simulink library "halout"  (R2021b)
settings: Solver=VariableStepAuto  StartTime=0.0  StopTime=10.0  RelTol=1e-3
undefined symbols (not defined in the file): C_TASK_5MS_S, FALSE, KHAL_CAN1FD1APS3E2E_flg, KHAL_CAN1FD1APS3TxReq_flg, KHAL_CAN1FD1VCU2E2E_flg, KHAL_CAN1FD1VCU2TxReq_flg, KHAL_CAN1FD1VCU3E2E_flg, KHAL_CAN1FD1VCU3TxReq_flg, KHAL_CAN1TxReq_flg, KHAL_CAN1VMCFCM1E2E_flg, KHAL_CAN1VMCFCM1TxReq_flg, KHAL_CAN2TxReq_flg, KHAL_CAN3FD3VCU1toNIDECTxReq_flg, KHAL_CAN3FD3VCU1TxReq_flg, KHAL_CAN3FD3VCU2E2E_flg, KHAL_CAN3FD3VCU2toNIDECE2E_flg, KHAL_CAN3FD3VCU2toNIDECTxReq_flg, KHAL_CAN3FD3VCU2TxReq_flg, KHAL_CAN3TxReq_flg, KHAL_CAN4FD4CE1000E2E_flg, KHAL_CAN4FD4CE1000TxReq_flg, KHAL_CAN4TxReq_flg, KHAL_CAN5TxReq_flg, KHAL_CAN6FD6APS3E2E_flg, KHAL_CAN6FD6APS3TxReq_flg, KHAL_CAN6FD6VCU2E2E_flg, KHAL_CAN6FD6VCU2TxReq_flg, KHAL_CAN6TxReq_flg, ONE_INT, TRUE, ZERO_INT
libraries: FVT_lib x500, simulink x235
(part 18 of 25)

== system halout/HAL_OUT/CAN2/FD2_CE200_1_0x435/LFWheelPress ==
  LFWheelPress : Inport
  Data Type Conversion : DataTypeConversion  OutDataTypeStr=uint8  RndMeth=Round
  CAN2_LFWheelPress : Outport
  wires:
  Data Type Conversion/1 -> CAN2_LFWheelPress/1
  LFWheelPress/1 -> Data Type Conversion/1

== system halout/HAL_OUT/CAN2/FD2_CE200_1_0x435/LFWheelShield ==
  LFWheelShield : Inport
  Data Type Conversion : DataTypeConversion  OutDataTypeStr=uint8  RndMeth=Round
  CAN2_LFWheelShield : Outport
  wires:
  Data Type Conversion/1 -> CAN2_LFWheelShield/1
  LFWheelShield/1 -> Data Type Conversion/1

== system halout/HAL_OUT/CAN2/FD2_CE200_1_0x435/LFWheelTemp ==
  LFWheelTemp : Inport
  Data Type Conversion : DataTypeConversion  OutDataTypeStr=uint8  RndMeth=Round
  convert_out : FVT_lib/hal/convert_out  gain=1  offset=-40
  CAN2_LFWheelTemp : Outport
  wires:
  Data Type Conversion/1 -> CAN2_LFWheelTemp/1
  convert_out/1 -> Data Type Conversion/1
  LFWheelTemp/1 -> convert_out/1

== system halout/HAL_OUT/CAN2/FD2_CE200_1_0x435/LFWheelTmpIndi ==
  LFWheelTmpIndi : Inport
  Data Type Conversion : DataTypeConversion  OutDataTypeStr=uint8  RndMeth=Round
  CAN2_LFWheelTmpIndi : Outport
  wires:
  Data Type Conversion/1 -> CAN2_LFWheelTmpIndi/1
  LFWheelTmpIndi/1 -> Data Type Conversion/1

== system halout/HAL_OUT/CAN2/FD2_CE200_1_0x435/LRBatWarn ==
  LRBatWarn : Inport
  Data Type Conversion : DataTypeConversion  OutDataTypeStr=uint8  RndMeth=Round
  CAN2_LRBatWarn : Outport
  wires:
  Data Type Conversion/1 -> CAN2_LRBatWarn/1
  LRBatWarn/1 -> Data Type Conversion/1

== system halout/HAL_OUT/CAN2/FD2_CE200_1_0x435/LRPressIndi ==
  LRPressIndi : Inport
  Data Type Conversion : DataTypeConversion  OutDataTypeStr=uint8  RndMeth=Round
  CAN2_LRPressIndi : Outport
  wires:
  Data Type Conversion/1 -> CAN2_LRPressIndi/1
  LRPressIndi/1 -> Data Type Conversion/1

== system halout/HAL_OUT/CAN2/FD2_CE200_1_0x435/LRSensorFail ==
  LRSensorFail : Inport
  Data Type Conversion : DataTypeConversion  OutDataTypeStr=uint8  RndMeth=Round
  CAN2_LRSensorFail : Outport
  wires:
  Data Type Conversion/1 -> CAN2_LRSensorFail/1
  LRSensorFail/1 -> Data Type Conversion/1

== system halout/HAL_OUT/CAN2/FD2_CE200_1_0x435/LRWheelDebug ==
  LRWheelDebug : Inport
  Data Type Conversion : DataTypeConversion  OutDataTypeStr=uint8  RndMeth=Round
  CAN2_LRWheelDebug : Outport
  wires:
  Data Type Conversion/1 -> CAN2_LRWheelDebug/1
  LRWheelDebug/1 -> Data Type Conversion/1

== system halout/HAL_OUT/CAN2/FD2_CE200_1_0x435/LRWheelPSW ==
  LRWheelPSW : Inport
  Data Type Conversion : DataTypeConversion  OutDataTypeStr=uint8  RndMeth=Round
  CAN2_LRWheelPSW : Outport
  wires:
  Data Type Conversion/1 -> CAN2_LRWheelPSW/1
  LRWheelPSW/1 -> Data Type Conversion/1

== system halout/HAL_OUT/CAN2/FD2_CE200_1_0x435/LRWheelPress ==
  LRWheelPress : Inport
  Data Type Conversion : DataTypeConversion  OutDataTypeStr=uint8  RndMeth=Round
  CAN2_LRWheelPress : Outport
  wires:
  Data Type Conversion/1 -> CAN2_LRWheelPress/1
  LRWheelPress/1 -> Data Type Conversion/1

== system halout/HAL_OUT/CAN2/FD2_CE200_1_0x435/LRWheelShield ==
  LRWheelShield : Inport
  Data Type Conversion : DataTypeConversion  OutDataTypeStr=uint8  RndMeth=Round
  CAN2_LRWheelShield : Outport
  wires:
  Data Type Conversion/1 -> CAN2_LRWheelShield/1
  LRWheelShield/1 -> Data Type Conversion/1

== system halout/HAL_OUT/CAN2/FD2_CE200_1_0x435/LRWheelTemp ==
  LRWheelTemp : Inport
  Data Type Conversion : DataTypeConversion  OutDataTypeStr=uint8  RndMeth=Round
  convert_out : FVT_lib/hal/convert_out  gain=1  offset=-40
  CAN2_LRWheelTemp : Outport
  wires:
  Data Type Conversion/1 -> CAN2_LRWheelTemp/1
  convert_out/1 -> Data Type Conversion/1
  LRWheelTemp/1 -> convert_out/1

== system halout/HAL_OUT/CAN2/FD2_CE200_1_0x435/LRWheelTmpIndi ==
  LRWheelTmpIndi : Inport
  Data Type Conversion : DataTypeConversion  OutDataTypeStr=uint8  RndMeth=Round
  CAN2_LRWheelTmpIndi : Outport
  wires:
  Data Type Conversion/1 -> CAN2_LRWheelTmpIndi/1
  LRWheelTmpIndi/1 -> Data Type Conversion/1

== system halout/HAL_OUT/CAN2/FD2_CE200_1_0x435/RFBatWarn ==
  RFBatWarn : Inport
  Data Type Conversion : DataTypeConversion  OutDataTypeStr=uint8  RndMeth=Round
  CAN2_RFBatWarn : Outport
  wires:
  Data Type Conversion/1 -> CAN2_RFBatWarn/1
  RFBatWarn/1 -> Data Type Conversion/1

== system halout/HAL_OUT/CAN2/FD2_CE200_1_0x435/RFPressIndi ==
  RFPressIndi : Inport
  Data Type Conversion : DataTypeConversion  OutDataTypeStr=uint8  RndMeth=Round
  CAN2_RFPressIndi : Outport
  wires:
  Data Type Conversion/1 -> CAN2_RFPressIndi/1
  RFPressIndi/1 -> Data Type Conversion/1

== system halout/HAL_OUT/CAN2/FD2_CE200_1_0x435/RFSensorFail ==
  RFSensorFail : Inport
  Data Type Conversion : DataTypeConversion  OutDataTypeStr=uint8  RndMeth=Round
  CAN2_RFSensorFail : Outport
  wires:
  Data Type Conversion/1 -> CAN2_RFSensorFail/1
  RFSensorFail/1 -> Data Type Conversion/1

== system halout/HAL_OUT/CAN2/FD2_CE200_1_0x435/RFWheelDebug ==
  RFWheelDebug : Inport
  Data Type Conversion : DataTypeConversion  OutDataTypeStr=uint8  RndMeth=Round
  CAN2_RFWheelDebug : Outport
  wires:
  Data Type Conversion/1 -> CAN2_RFWheelDebug/1
  RFWheelDebug/1 -> Data Type Conversion/1

== system halout/HAL_OUT/CAN2/FD2_CE200_1_0x435/RFWheelPSW ==
  RFWheelPSW : Inport
  Data Type Conversion : DataTypeConversion  OutDataTypeStr=uint8  RndMeth=Round
  CAN2_RFWheelPSW : Outport
  wires:
  Data Type Conversion/1 -> CAN2_RFWheelPSW/1
  RFWheelPSW/1 -> Data Type Conversion/1

== system halout/HAL_OUT/CAN2/FD2_CE200_1_0x435/RFWheelPress ==
  RFWheelPress : Inport
  Data Type Conversion : DataTypeConversion  OutDataTypeStr=uint8  RndMeth=Round
  CAN2_RFWheelPress : Outport
  wires:
  Data Type Conversion/1 -> CAN2_RFWheelPress/1
  RFWheelPress/1 -> Data Type Conversion/1

== system halout/HAL_OUT/CAN2/FD2_CE200_1_0x435/RFWheelShield ==
  RFWheelShield : Inport
  Data Type Conversion : DataTypeConversion  OutDataTypeStr=uint8  RndMeth=Round
  CAN2_RFWheelShield : Outport
  wires:
  Data Type Conversion/1 -> CAN2_RFWheelShield/1
  RFWheelShield/1 -> Data Type Conversion/1

== system halout/HAL_OUT/CAN2/FD2_CE200_1_0x435/RFWheelTemp ==
  RFWheelTemp : Inport
  Data Type Conversion : DataTypeConversion  OutDataTypeStr=uint8  RndMeth=Round
  convert_out : FVT_lib/hal/convert_out  gain=1  offset=-40
  CAN2_RFWheelTemp : Outport
  wires:
  Data Type Conversion/1 -> CAN2_RFWheelTemp/1
  convert_out/1 -> Data Type Conversion/1
  RFWheelTemp/1 -> convert_out/1

== system halout/HAL_OUT/CAN2/FD2_CE200_1_0x435/RFWheelTmpIndi ==
  RFWheelTmpIndi : Inport
  Data Type Conversion : DataTypeConversion  OutDataTypeStr=uint8  RndMeth=Round
  CAN2_RFWheelTmpIndi : Outport
  wires:
  Data Type Conversion/1 -> CAN2_RFWheelTmpIndi/1
  RFWheelTmpIndi/1 -> Data Type Conversion/1

== system halout/HAL_OUT/CAN2/FD2_CE200_1_0x435/RRBatWarn ==
  RRBatWarn : Inport
  Data Type Conversion : DataTypeConversion  OutDataTypeStr=uint8  RndMeth=Round
  CAN2_RRBatWarn : Outport
  wires:
  Data Type Conversion/1 -> CAN2_RRBatWarn/1
  RRBatWarn/1 -> Data Type Conversion/1

== system halout/HAL_OUT/CAN2/FD2_CE200_1_0x435/RRPressIndi ==
  RRPressIndi : Inport
  Data Type Conversion : DataTypeConversion  OutDataTypeStr=uint8  RndMeth=Round
  CAN2_RRPressIndi : Outport
  wires:
  Data Type Conversion/1 -> CAN2_RRPressIndi/1
  RRPressIndi/1 -> Data Type Conversion/1

== system halout/HAL_OUT/CAN2/FD2_CE200_1_0x435/RRSensorFail ==
  RRSensorFail : Inport
  Data Type Conversion : DataTypeConversion  OutDataTypeStr=uint8  RndMeth=Round
  CAN2_RRSensorFail : Outport
  wires:
  Data Type Conversion/1 -> CAN2_RRSensorFail/1
  RRSensorFail/1 -> Data Type Conversion/1

== system halout/HAL_OUT/CAN2/FD2_CE200_1_0x435/RRWheelDebug ==
  RRWheelDebug : Inport
  Data Type Conversion : DataTypeConversion  OutDataTypeStr=uint8  RndMeth=Round
  CAN2_RRWheelDebug : Outport
  wires:
  Data Type Conversion/1 -> CAN2_RRWheelDebug/1
  RRWheelDebug/1 -> Data Type Conversion/1

== system halout/HAL_OUT/CAN2/FD2_CE200_1_0x435/RRWheelPSW ==
  RRWheelPSW : Inport
  Data Type Conversion : DataTypeConversion  OutDataTypeStr=uint8  RndMeth=Round
  CAN2_RRWheelPSW : Outport
  wires:
  Data Type Conversion/1 -> CAN2_RRWheelPSW/1
  RRWheelPSW/1 -> Data Type Conversion/1

== system halout/HAL_OUT/CAN2/FD2_CE200_1_0x435/RRWheelPress ==
  RRWheelPress : Inport
  Data Type Conversion : DataTypeConversion  OutDataTypeStr=uint8  RndMeth=Round
  CAN2_RRWheelPress : Outport
  wires:
  Data Type Conversion/1 -> CAN2_RRWheelPress/1
  RRWheelPress/1 -> Data Type Conversion/1

== system halout/HAL_OUT/CAN2/FD2_CE200_1_0x435/RRWheelShield ==
  RRWheelShield : Inport
  Data Type Conversion : DataTypeConversion  OutDataTypeStr=uint8  RndMeth=Round
  CAN2_RRWheelShield : Outport
  wires:
  Data Type Conversion/1 -> CAN2_RRWheelShield/1
  RRWheelShield/1 -> Data Type Conversion/1

== system halout/HAL_OUT/CAN2/FD2_CE200_1_0x435/RRWheelTemp ==
  RRWheelTemp : Inport
  Data Type Conversion : DataTypeConversion  OutDataTypeStr=uint8  RndMeth=Round
  convert_out : FVT_lib/hal/convert_out  gain=1  offset=-40
  CAN2_RRWheelTemp : Outport
  wires:
  Data Type Conversion/1 -> CAN2_RRWheelTemp/1
  convert_out/1 -> Data Type Conversion/1
  RRWheelTemp/1 -> convert_out/1

== system halout/HAL_OUT/CAN2/FD2_CE200_1_0x435/RRWheelTmpIndi ==
  RRWheelTmpIndi : Inport
  Data Type Conversion : DataTypeConversion  OutDataTypeStr=uint8  RndMeth=Round
  CAN2_RRWheelTmpIndi : Outport
  wires:
  Data Type Conversion/1 -> CAN2_RRWheelTmpIndi/1
  RRWheelTmpIndi/1 -> Data Type Conversion/1

== system halout/HAL_OUT/CAN2/FD2_CE200_1_0x435/TPMSCaliButtAllow ==
  TPMSCaliButtAllow : Inport
  Data Type Conversion : DataTypeConversion  OutDataTypeStr=uint8  RndMeth=Round
  CAN2_TPMS_Cali_Butt_Allow : Outport
  wires:
  Data Type Conversion/1 -> CAN2_TPMS_Cali_Butt_Allow/1
  TPMSCaliButtAllow/1 -> Data Type Conversion/1

== system halout/HAL_OUT/CAN2/FD2_CE200_1_0x435/TPMSResButtAllow ==
  TPMSResButtAllow : Inport
  Data Type Conversion : DataTypeConversion  OutDataTypeStr=uint8  RndMeth=Round
  CAN2_TPMS_Res_Butt_Allow : Outport
  wires:
  Data Type Conversion/1 -> CAN2_TPMS_Res_Butt_Allow/1
  TPMSResButtAllow/1 -> Data Type Conversion/1

== system halout/HAL_OUT/CAN2/FD2_CE200_1_0x435/TPMSWarnIndi ==
  TPMSWarnIndi : Inport
  Data Type Conversion : DataTypeConversion  OutDataTypeStr=uint8  RndMeth=Round
  CAN2_TPMSWarnIndi : Outport
  wires:
  Data Type Conversion/1 -> CAN2_TPMSWarnIndi/1
  TPMSWarnIndi/1 -> Data Type Conversion/1

== system halout/HAL_OUT/CAN2/FD2_Version_0x3C3/FUSIONHWVer1 ==
  FUSIONHWVer1 : Inport
  Data Type Conversion : DataTypeConversion  OutDataTypeStr=uint8  RndMeth=Round
  CAN2_FUSION_HW_Ver1 : Outport
  wires:
  Data Type Conversion/1 -> CAN2_FUSION_HW_Ver1/1
  FUSIONHWVer1/1 -> Data Type Conversion/1

== system halout/HAL_OUT/CAN2/FD2_Version_0x3C3/FUSIONHWVer2 ==
  FUSIONHWVer2 : Inport
  Data Type Conversion : DataTypeConversion  OutDataTypeStr=uint8  RndMeth=Round
  CAN2_FUSION_HW_Ver2 : Outport
  wires:
  Data Type Conversion/1 -> CAN2_FUSION_HW_Ver2/1
  FUSIONHWVer2/1 -> Data Type Conversion/1

== system halout/HAL_OUT/CAN2/FD2_Version_0x3C3/FUSIONHWVer3 ==
  FUSIONHWVer3 : Inport
  Data Type Conversion : DataTypeConversion  OutDataTypeStr=uint8  RndMeth=Round
  CAN2_FUSION_HW_Ver3 : Outport
  wires:
  Data Type Conversion/1 -> CAN2_FUSION_HW_Ver3/1
  FUSIONHWVer3/1 -> Data Type Conversion/1

== system halout/HAL_OUT/CAN2/FD2_Version_0x3C3/FUSIONSWCarModel1 ==
  FUSIONSWCarModel1 : Inport
  Data Type Conversion : DataTypeConversion  OutDataTypeStr=uint8  RndMeth=Round
  CAN2_FUSION_SW_CarModel1 : Outport
  wires:
  Data Type Conversion/1 -> CAN2_FUSION_SW_CarModel1/1
  FUSIONSWCarModel1/1 -> Data Type Conversion/1

== system halout/HAL_OUT/CAN2/FD2_Version_0x3C3/FUSIONSWCarModel2 ==
  FUSIONSWCarModel2 : Inport
  Data Type Conversion : DataTypeConversion  OutDataTypeStr=uint8  RndMeth=Round
  CAN2_FUSION_SW_CarModel2 : Outport
  wires:
  Data Type Conversion/1 -> CAN2_FUSION_SW_CarModel2/1
  FUSIONSWCarModel2/1 -> Data Type Conversion/1

== system halout/HAL_OUT/CAN2/FD2_Version_0x3C3/FUSIONSWCarModel3 ==
  FUSIONSWCarModel3 : Inport
  Data Type Conversion : DataTypeConversion  OutDataTypeStr=uint8  RndMeth=Round
  CAN2_FUSION_SW_CarModel3 : Outport
  wires:
  Data Type Conversion/1 -> CAN2_FUSION_SW_CarModel3/1
  FUSIONSWCarModel3/1 -> Data Type Conversion/1

== system halout/HAL_OUT/CAN2/FD2_Version_0x3C3/FUSIONSWController1 ==
  FUSIONSWController1 : Inport
  Data Type Conversion : DataTypeConversion  OutDataTypeStr=uint8  RndMeth=Round
  CAN2_FUSION_SW_Controller1 : Outport
  wires:
  Data Type Conversion/1 -> CAN2_FUSION_SW_Controller1/1
  FUSIONSWController1/1 -> Data Type Conversion/1

== system halout/HAL_OUT/CAN2/FD2_Version_0x3C3/FUSIONSWController2 ==
  FUSIONSWController2 : Inport
  Data Type Conversion : DataTypeConversion  OutDataTypeStr=uint8  RndMeth=Round
  CAN2_FUSION_SW_Controller2 : Outport
  wires:
  Data Type Conversion/1 -> CAN2_FUSION_SW_Controller2/1
  FUSIONSWController2/1 -> Data Type Conversion/1

== system halout/HAL_OUT/CAN2/FD2_Version_0x3C3/FUSIONSWCountry1 ==
  FUSIONSWCountry1 : Inport
  Data Type Conversion : DataTypeConversion  OutDataTypeStr=uint8  RndMeth=Round
  CAN2_FUSION_SW_Country1 : Outport
  wires:
  Data Type Conversion/1 -> CAN2_FUSION_SW_Country1/1
  FUSIONSWCountry1/1 -> Data Type Conversion/1

== system halout/HAL_OUT/CAN2/FD2_Version_0x3C3/FUSIONSWCountry2 ==
  FUSIONSWCountry2 : Inport
  Data Type Conversion : DataTypeConversion  OutDataTypeStr=uint8  RndMeth=Round
  CAN2_FUSION_SW_Country2 : Outport
  wires:
  Data Type Conversion/1 -> CAN2_FUSION_SW_Country2/1
  FUSIONSWCountry2/1 -> Data Type Conversion/1

== system halout/HAL_OUT/CAN2/FD2_Version_0x3C3/FUSIONSWECUGen1 ==
  FUSIONSWECUGen1 : Inport
  Data Type Conversion : DataTypeConversion  OutDataTypeStr=uint8  RndMeth=Round
  CAN2_FUSION_SW_ECUGen1 : Outport
  wires:
  Data Type Conversion/1 -> CAN2_FUSION_SW_ECUGen1/1
  FUSIONSWECUGen1/1 -> Data Type Conversion/1

== system halout/HAL_OUT/CAN2/FD2_Version_0x3C3/FUSIONSWECUGen2 ==
  FUSIONSWECUGen2 : Inport
  Data Type Conversion : DataTypeConversion  OutDataTypeStr=uint8  RndMeth=Round
  CAN2_FUSION_SW_ECUGen2 : Outport
  wires:
  Data Type Conversion/1 -> CAN2_FUSION_SW_ECUGen2/1
  FUSIONSWECUGen2/1 -> Data Type Conversion/1

== system halout/HAL_OUT/CAN2/FD2_Version_0x3C3/FUSIONSWMajor1 ==
  FUSIONSWMajor1 : Inport
  Data Type Conversion : DataTypeConversion  OutDataTypeStr=uint8  RndMeth=Round
  CAN2_FUSION_SW_Major1 : Outport
  wires:
  Data Type Conversion/1 -> CAN2_FUSION_SW_Major1/1
  FUSIONSWMajor1/1 -> Data Type Conversion/1

== system halout/HAL_OUT/CAN2/FD2_Version_0x3C3/FUSIONSWMajor2 ==
  FUSIONSWMajor2 : Inport
  Data Type Conversion : DataTypeConversion  OutDataTypeStr=uint8  RndMeth=Round
  CAN2_FUSION_SW_Major2 : Outport
  wires:
  Data Type Conversion/1 -> CAN2_FUSION_SW_Major2/1
  FUSIONSWMajor2/1 -> Data Type Conversion/1

== system halout/HAL_OUT/CAN2/FD2_Version_0x3C3/FUSIONSWMinor1 ==
  FUSIONSWMinor1 : Inport
  Data Type Conversion : DataTypeConversion  OutDataTypeStr=uint8  RndMeth=Round
  CAN2_FUSION_SW_Minor1 : Outport
  wires:
  Data Type Conversion/1 -> CAN2_FUSION_SW_Minor1/1
  FUSIONSWMinor1/1 -> Data Type Conversion/1

== system halout/HAL_OUT/CAN2/FD2_Version_0x3C3/FUSIONSWMinor2 ==
  FUSIONSWMinor2 : Inport
  Data Type Conversion : DataTypeConversion  OutDataTypeStr=uint8  RndMeth=Round
  CAN2_FUSION_SW_Minor2 : Outport
  wires:
  Data Type Conversion/1 -> CAN2_FUSION_SW_Minor2/1
  FUSIONSWMinor2/1 -> Data Type Conversion/1

== system halout/HAL_OUT/CAN2/FD2_Version_0x3C3/FUSIONSWPatch1 ==
  FUSIONSWPatch1 : Inport
  Data Type Conversion : DataTypeConversion  OutDataTypeStr=uint8  RndMeth=Round
  CAN2_FUSION_SW_Patch1 : Outport
  wires:
  Data Type Conversion/1 -> CAN2_FUSION_SW_Patch1/1
  FUSIONSWPatch1/1 -> Data Type Conversion/1

== system halout/HAL_OUT/CAN2/FD2_Version_0x3C3/FUSIONSWPatch2 ==
  FUSIONSWPatch2 : Inport
  Data Type Conversion : DataTypeConversion  OutDataTypeStr=uint8  RndMeth=Round
  CAN2_FUSION_SW_Patch2 : Outport
  wires:
  Data Type Conversion/1 -> CAN2_FUSION_SW_Patch2/1
  FUSIONSWPatch2/1 -> Data Type Conversion/1

== system halout/HAL_OUT/CAN2/FD2_Version_0x3C3/FUSIONSWSHA1 ==
  FUSIONSWSHA1 : Inport
  Data Type Conversion : DataTypeConversion  OutDataTypeStr=uint8  RndMeth=Round
  CAN2_FUSION_SW_SHA1 : Outport
  wires:
  Data Type Conversion/1 -> CAN2_FUSION_SW_SHA1/1
  FUSIONSWSHA1/1 -> Data Type Conversion/1

== system halout/HAL_OUT/CAN2/FD2_Version_0x3C3/FUSIONSWSHA2 ==
  FUSIONSWSHA2 : Inport
  Data Type Conversion : DataTypeConversion  OutDataTypeStr=uint8  RndMeth=Round
  CAN2_FUSION_SW_SHA2 : Outport
  wires:
  Data Type Conversion/1 -> CAN2_FUSION_SW_SHA2/1
  FUSIONSWSHA2/1 -> Data Type Conversion/1

== system halout/HAL_OUT/CAN2/FD2_Version_0x3C3/FUSIONSWSHA3 ==
  FUSIONSWSHA3 : Inport
  Data Type Conversion : DataTypeConversion  OutDataTypeStr=uint8  RndMeth=Round
  CAN2_FUSION_SW_SHA3 : Outport
  wires:
  Data Type Conversion/1 -> CAN2_FUSION_SW_SHA3/1
  FUSIONSWSHA3/1 -> Data Type Conversion/1

== system halout/HAL_OUT/CAN2/FD2_Version_0x3C3/FUSIONSWSHA4 ==
  FUSIONSWSHA4 : Inport
  Data Type Conversion : DataTypeConversion  OutDataTypeStr=uint8  RndMeth=Round
  CAN2_FUSION_SW_SHA4 : Outport
  wires:
  Data Type Conversion/1 -> CAN2_FUSION_SW_SHA4/1
  FUSIONSWSHA4/1 -> Data Type Conversion/1

== system halout/HAL_OUT/CAN2/FD2_Version_0x3C3/FUSIONSWSHA5 ==
  FUSIONSWSHA5 : Inport
  Data Type Conversion : DataTypeConversion  OutDataTypeStr=uint8  RndMeth=Round
  CAN2_FUSION_SW_SHA5 : Outport
  wires:
  Data Type Conversion/1 -> CAN2_FUSION_SW_SHA5/1
  FUSIONSWSHA5/1 -> Data Type Conversion/1

== system halout/HAL_OUT/CAN2/FD2_Version_0x3C3/FUSIONSWSHA6 ==
  FUSIONSWSHA6 : Inport
  Data Type Conversion : DataTypeConversion  OutDataTypeStr=uint8  RndMeth=Round
  CAN2_FUSION_SW_SHA6 : Outport
  wires:
  Data Type Conversion/1 -> CAN2_FUSION_SW_SHA6/1
  FUSIONSWSHA6/1 -> Data Type Conversion/1

== system halout/HAL_OUT/CAN2/FD2_Version_0x3C3/FUSIONSWSHA7 ==
  FUSIONSWSHA7 : Inport
  Data Type Conversion : DataTypeConversion  OutDataTypeStr=uint8  RndMeth=Round
  CAN2_FUSION_SW_SHA7 : Outport
  wires:
  Data Type Conversion/1 -> CAN2_FUSION_SW_SHA7/1
  FUSIONSWSHA7/1 -> Data Type Conversion/1

== system halout/HAL_OUT/CAN2/FD2_Version_0x3C3/FUSIONSWSHA8 ==
  FUSIONSWSHA8 : Inport
  Data Type Conversion : DataTypeConversion  OutDataTypeStr=uint8  RndMeth=Round
  CAN2_FUSION_SW_SHA8 : Outport
  wires:
  Data Type Conversion/1 -> CAN2_FUSION_SW_SHA8/1
  FUSIONSWSHA8/1 -> Data Type Conversion/1

== system halout/HAL_OUT/CAN2/FD2_Version_0x3C3/FUSIONSWVar1 ==
  FUSIONSWVar1 : Inport
  Data Type Conversion : DataTypeConversion  OutDataTypeStr=uint8  RndMeth=Round
  CAN2_FUSION_SW_Var1 : Outport
  wires:
  Data Type Conversion/1 -> CAN2_FUSION_SW_Var1/1
  FUSIONSWVar1/1 -> Data Type Conversion/1

== system halout/HAL_OUT/CAN2/FD2_Version_0x3C3/FUSIONSWVar2 ==
  FUSIONSWVar2 : Inport
  Data Type Conversion : DataTypeConversion  OutDataTypeStr=uint8  RndMeth=Round
  CAN2_FUSION_SW_Var2 : Outport
  wires:
  Data Type Conversion/1 -> CAN2_FUSION_SW_Var2/1
  FUSIONSWVar2/1 -> Data Type Conversion/1

== system halout/HAL_OUT/CAN2/FD2_Version_0x3C3/FUSIONSWVar3 ==
  FUSIONSWVar3 : Inport
  Data Type Conversion : DataTypeConversion  OutDataTypeStr=uint8  RndMeth=Round
  CAN2_FUSION_SW_Var3 : Outport
  wires:
  Data Type Conversion/1 -> CAN2_FUSION_SW_Var3/1
  FUSIONSWVar3/1 -> Data Type Conversion/1

== system halout/HAL_OUT/CAN2/FD2_Version_0x3C3/FUSIONSWVar4 ==
  FUSIONSWVar4 : Inport
  Data Type Conversion : DataTypeConversion  OutDataTypeStr=uint8  RndMeth=Round
  CAN2_FUSION_SW_Var4 : Outport
  wires:
  Data Type Conversion/1 -> CAN2_FUSION_SW_Var4/1
  FUSIONSWVar4/1 -> Data Type Conversion/1

== system halout/HAL_OUT/CAN2/FD2_Version_0x3C3/FUSIONSWVar5 ==
  FUSIONSWVar5 : Inport
  Data Type Conversion : DataTypeConversion  OutDataTypeStr=uint8  RndMeth=Round
  CAN2_FUSION_SW_Var5 : Outport
  wires:
  Data Type Conversion/1 -> CAN2_FUSION_SW_Var5/1
  FUSIONSWVar5/1 -> Data Type Conversion/1

== system halout/HAL_OUT/CAN2/FD2_Version_0x3C3/FUSIONSWchange1 ==
  FUSIONSWchange1 : Inport
  Data Type Conversion : DataTypeConversion  OutDataTypeStr=uint8  RndMeth=Round
  CAN2_FUSION_SW_change1 : Outport
  wires:
  Data Type Conversion/1 -> CAN2_FUSION_SW_change1/1
  FUSIONSWchange1/1 -> Data Type Conversion/1

== system halout/HAL_OUT/CAN2/FD2_Version_0x3C3/FUSIONSWchange2 ==
  FUSIONSWchange2 : Inport
  Data Type Conversion : DataTypeConversion  OutDataTypeStr=uint8  RndMeth=Round
  CAN2_FUSION_SW_change2 : Outport
  wires:
  Data Type Conversion/1 -> CAN2_FUSION_SW_change2/1
  FUSIONSWchange2/1 -> Data Type Conversion/1

== system halout/HAL_OUT/CAN2/FD2_Version_0x3C3/FUSIONSWdash1 ==
  FUSIONSWdash1 : Inport
  Data Type Conversion : DataTypeConversion  OutDataTypeStr=uint8  RndMeth=Round
  CAN2_FUSION_SW_dash1 : Outport
  wires:
  Data Type Conversion/1 -> CAN2_FUSION_SW_dash1/1
  FUSIONSWdash1/1 -> Data Type Conversion/1

== system halout/HAL_OUT/CAN2/FD2_Version_0x3C3/FUSIONSWdash2 ==
  FUSIONSWdash2 : Inport
  Data Type Conversion : DataTypeConversion  OutDataTypeStr=uint8  RndMeth=Round
  CAN2_FUSION_SW_dash2 : Outport
  wires:
  Data Type Conversion/1 -> CAN2_FUSION_SW_dash2/1
  FUSIONSWdash2/1 -> Data Type Conversion/1

== system halout/HAL_OUT/CAN2/GW2_CE100_0_0x1C2/FDCBCMDimSw ==
  FDCBCMDimSw : Inport
  Data Type Conversion : DataTypeConversion  OutDataTypeStr=uint8  RndMeth=Round
  CAN2_FDC_BCM_DimSw : Outport
  wires:
  Data Type Conversion/1 -> CAN2_FDC_BCM_DimSw/1
  FDCBCMDimSw/1 -> Data Type Conversion/1

== system halout/HAL_OUT/CAN2/GW2_CE100_0_0x1C2/FDCBCMFWipSwSta ==
  FDCBCMFWipSwSta : Inport
  Data Type Conversion : DataTypeConversion  OutDataTypeStr=uint8  RndMeth=Round
  CAN2_FDC_BCM_FWipSw_Sta : Outport
  wires:
  Data Type Conversion/1 -> CAN2_FDC_BCM_FWipSw_Sta/1
  FDCBCMFWipSwSta/1 -> Data Type Conversion/1

== system halout/HAL_OUT/CAN2/GW2_CE100_0_0x1C2/FDCBCMTurnSwSta ==
  FDCBCMTurnSwSta : Inport
  Data Type Conversion : DataTypeConversion  OutDataTypeStr=uint8  RndMeth=Round
  CAN2_FDC_BCM_TurnSw_Sta : Outport
  wires:
  Data Type Conversion/1 -> CAN2_FDC_BCM_TurnSw_Sta/1
  FDCBCMTurnSwSta/1 -> Data Type Conversion/1

== system halout/HAL_OUT/CAN3/FD3_BCM1_0x216/AllDoorSW ==
  AllDoorSW : Inport
  Data Type Conversion : DataTypeConversion  OutDataTypeStr=uint8  RndMeth=Round
  CAN3_AllDoorSW : Outport
  wires:
  Data Type Conversion/1 -> CAN3_AllDoorSW/1
  AllDoorSW/1 -> Data Type Conversion/1

== system halout/HAL_OUT/CAN3/FD3_BCM1_0x216/AntiTheftSeatFold ==
  AntiTheftSeatFold : Inport
  Data Type Conversion : DataTypeConversion  OutDataTypeStr=uint8  RndMeth=Round
  CAN3_AntiTheftSeatFold : Outport
  wires:
  Data Type Conversion/1 -> CAN3_AntiTheftSeatFold/1
  AntiTheftSeatFold/1 -> Data Type Conversion/1

== system halout/HAL_OUT/CAN3/FD3_BCM1_0x216/AntitheftSta ==
  AntitheftSta : Inport
  Data Type Conversion : DataTypeConversion  OutDataTypeStr=uint8  RndMeth=Round
  CAN3_AntitheftSta : Outport
  wires:
  Data Type Conversion/1 -> CAN3_AntitheftSta/1
  AntitheftSta/1 -> Data Type Conversion/1

== system halout/HAL_OUT/CAN3/FD3_BCM1_0x216/BCMBuzzerReq ==
  BCMBuzzerReq : Inport
  Data Type Conversion : DataTypeConversion  OutDataTypeStr=uint8  RndMeth=Round
  CAN3_BCM_Buzzer_Req : Outport
  wires:
  Data Type Conversion/1 -> CAN3_BCM_Buzzer_Req/1
  BCMBuzzerReq/1 -> Data Type Conversion/1

== system halout/HAL_OUT/CAN3/FD3_BCM1_0x216/BCMDoorLockSta ==
  BCMDoorLockSta : Inport
  Data Type Conversion : DataTypeConversion  OutDataTypeStr=uint8  RndMeth=Round
  CAN3_BCM_DoorLock_Sta : Outport
  wires:
  Data Type Conversion/1 -> CAN3_BCM_DoorLock_Sta/1
  BCMDoorLockSta/1 -> Data Type Conversion/1

== system halout/HAL_OUT/CAN3/FD3_BCM1_0x216/BrakeLamp ==
  BrakeLamp : Inport
  Data Type Conversion : DataTypeConversion  OutDataTypeStr=uint8  RndMeth=Round
  CAN3_BrakeLamp : Outport
  wires:
  Data Type Conversion/1 -> CAN3_BrakeLamp/1
  BrakeLamp/1 -> Data Type Conversion/1

== system halout/HAL_OUT/CAN3/FD3_BCM1_0x216/CTDCtrl ==
  CTDCtrl : Inport
  Data Type Conversion : DataTypeConversion  OutDataTypeStr=uint8  RndMeth=Round
  CAN3_CTDCtrl : Outport
  wires:
  Data Type Conversion/1 -> CAN3_CTDCtrl/1
  CTDCtrl/1 -> Data Type Conversion/1

== system halout/HAL_OUT/CAN3/FD3_BCM1_0x216/CTDLockSW ==
  CTDLockSW : Inport
  Data Type Conversion : DataTypeConversion  OutDataTypeStr=uint8  RndMeth=Round
  CAN3_CTDLockSW : Outport
  wires:
  Data Type Conversion/1 -> CAN3_CTDLockSW/1
  CTDLockSW/1 -> Data Type Conversion/1

== system halout/HAL_OUT/CAN3/FD3_BCM1_0x216/CTDUnlockSW ==
  CTDUnlockSW : Inport
  Data Type Conversion : DataTypeConversion  OutDataTypeStr=uint8  RndMeth=Round
  CAN3_CTDUnlockSW : Outport
  wires:
  Data Type Conversion/1 -> CAN3_CTDUnlockSW/1
  CTDUnlockSW/1 -> Data Type Conversion/1

== system halout/HAL_OUT/CAN3/FD3_BCM1_0x216/CrashDetd ==
  CrashDetd : Inport
  Data Type Conversion : DataTypeConversion  OutDataTypeStr=uint8  RndMeth=Round
  CAN3_CrashDetd : Outport
  wires:
  Data Type Conversion/1 -> CAN3_CrashDetd/1
  CrashDetd/1 -> Data Type Conversion/1

== system halout/HAL_OUT/CAN3/FD3_BCM1_0x216/Dimmer ==
  Dimmer : Inport
  Data Type Conversion : DataTypeConversion  OutDataTypeStr=uint8  RndMeth=Round
  CAN3_Dimmer : Outport
  wires:
  Data Type Conversion/1 -> CAN3_Dimmer/1
  Dimmer/1 -> Data Type Conversion/1

== system halout/HAL_OUT/CAN3/FD3_BCM1_0x216/DimmerEN ==
  DimmerEN : Inport
  Data Type Conversion : DataTypeConversion  OutDataTypeStr=uint8  RndMeth=Round
  CAN3_DimmerEN : Outport
  wires:
  Data Type Conversion/1 -> CAN3_DimmerEN/1
  DimmerEN/1 -> Data Type Conversion/1

== system halout/HAL_OUT/CAN3/FD3_BCM1_0x216/DoorLockIND ==
  DoorLockIND : Inport
  Data Type Conversion : DataTypeConversion  OutDataTypeStr=uint8  RndMeth=Round
  CAN3_DoorLockIND : Outport
  wires:
  Data Type Conversion/1 -> CAN3_DoorLockIND/1
  DoorLockIND/1 -> Data Type Conversion/1

== system halout/HAL_OUT/CAN3/FD3_BCM1_0x216/DrDoorSW ==
  DrDoorSW : Inport
  Data Type Conversion : DataTypeConversion  OutDataTypeStr=uint8  RndMeth=Round
  CAN3_DrDoorSW : Outport
  wires:
  Data Type Conversion/1 -> CAN3_DrDoorSW/1
  DrDoorSW/1 -> Data Type Conversion/1

== system halout/HAL_OUT/CAN3/FD3_BCM1_0x216/FrChargingDoorCtrl ==
  FrChargingDoorCtrl : Inport
  Data Type Conversion : DataTypeConversion  OutDataTypeStr=uint8  RndMeth=Round
  CAN3_Fr_ChargingDoorCtrl : Outport
  wires:
  Data Type Conversion/1 -> CAN3_Fr_ChargingDoorCtrl/1
  FrChargingDoorCtrl/1 -> Data Type Conversion/1

== system halout/HAL_OUT/CAN3/FD3_BCM1_0x216/FrFogLamp ==
  FrFogLamp : Inport
  Data Type Conversion : DataTypeConversion  OutDataTypeStr=uint8  RndMeth=Round
  CAN3_Fr_FogLamp : Outport
  wires:
  Data Type Conversion/1 -> CAN3_Fr_FogLamp/1
  FrFogLamp/1 -> Data Type Conversion/1

== system halout/HAL_OUT/CAN3/FD3_BCM1_0x216/FrWiperH ==
  FrWiperH : Inport
  Data Type Conversion : DataTypeConversion  OutDataTypeStr=uint8  RndMeth=Round
  CAN3_Fr_Wiper_H : Outport
  wires:
  Data Type Conversion/1 -> CAN3_Fr_Wiper_H/1
  FrWiperH/1 -> Data Type Conversion/1

== system halout/HAL_OUT/CAN3/FD3_BCM1_0x216/FrWiperL ==
  FrWiperL : Inport
  Data Type Conversion : DataTypeConversion  OutDataTypeStr=uint8  RndMeth=Round
  CAN3_Fr_Wiper_L : Outport
  wires:
  Data Type Conversion/1 -> CAN3_Fr_Wiper_L/1
  FrWiperL/1 -> Data Type Conversion/1

== system halout/HAL_OUT/CAN3/FD3_BCM1_0x216/HBeam ==
  HBeam : Inport
  Data Type Conversion : DataTypeConversion  OutDataTypeStr=uint8  RndMeth=Round
  CAN3_H_Beam : Outport
  wires:
  Data Type Conversion/1 -> CAN3_H_Beam/1
  HBeam/1 -> Data Type Conversion/1

== system halout/HAL_OUT/CAN3/FD3_BCM1_0x216/HazardSW ==
  HazardSW : Inport
  Data Type Conversion : DataTypeConversion  OutDataTypeStr=uint8  RndMeth=Round
  CAN3_HazardSW : Outport
  wires:
  Data Type Conversion/1 -> CAN3_HazardSW/1
  HazardSW/1 -> Data Type Conversion/1

== system halout/HAL_OUT/CAN3/FD3_BCM1_0x216/HoodSW ==
  HoodSW : Inport
  Data Type Conversion : DataTypeConversion  OutDataTypeStr=uint8  RndMeth=Round
  CAN3_HoodSW : Outport
  wires:
  Data Type Conversion/1 -> CAN3_HoodSW/1
  HoodSW/1 -> Data Type Conversion/1

== system halout/HAL_OUT/CAN3/FD3_BCM1_0x216/HornCtrl ==
  HornCtrl : Inport
  Data Type Conversion : DataTypeConversion  OutDataTypeStr=uint8  RndMeth=Round
  CAN3_HornCtrl : Outport
  wires:
  Data Type Conversion/1 -> CAN3_HornCtrl/1
  HornCtrl/1 -> Data Type Conversion/1

== system halout/HAL_OUT/CAN3/FD3_BCM1_0x216/LAPMWdwEnable ==
  LAPMWdwEnable : Inport
  Data Type Conversion : DataTypeConversion  OutDataTypeStr=uint8  RndMeth=Round
  CAN3_L_APM_WdwEnable : Outport
  wires:
  Data Type Conversion/1 -> CAN3_L_APM_WdwEnable/1
  LAPMWdwEnable/1 -> Data Type Conversion/1

== system halout/HAL_OUT/CAN3/FD3_BCM1_0x216/LBSD ==
  LBSD : Inport
  Data Type Conversion : DataTypeConversion  OutDataTypeStr=uint8  RndMeth=Round
  CAN3_LBSD : Outport
  wires:
  Data Type Conversion/1 -> CAN3_LBSD/1
  LBSD/1 -> Data Type Conversion/1

== system halout/HAL_OUT/CAN3/FD3_BCM1_0x216/LBeam ==
  LBeam : Inport
  Data Type Conversion : DataTypeConversion  OutDataTypeStr=uint8  RndMeth=Round
  CAN3_L_Beam : Outport
  wires:
  Data Type Conversion/1 -> CAN3_L_Beam/1
  LBeam/1 -> Data Type Conversion/1

== system halout/HAL_OUT/CAN3/FD3_BCM1_0x216/LDRL ==
  LDRL : Inport
  Data Type Conversion : DataTypeConversion  OutDataTypeStr=uint8  RndMeth=Round
  CAN3_LDRL : Outport
  wires:
  Data Type Conversion/1 -> CAN3_LDRL/1
  LDRL/1 -> Data Type Conversion/1

== system halout/HAL_OUT/CAN3/FD3_BCM1_0x216/LTurnLP ==
  LTurnLP : Inport
  Data Type Conversion : DataTypeConversion  OutDataTypeStr=uint8  RndMeth=Round
  CAN3_LTurnLP : Outport
  wires:
  Data Type Conversion/1 -> CAN3_LTurnLP/1
  LTurnLP/1 -> Data Type Conversion/1

== system halout/HAL_OUT/CAN3/FD3_BCM1_0x216/LockSetting ==
  LockSetting : Inport
  Data Type Conversion : DataTypeConversion  OutDataTypeStr=uint8  RndMeth=Round
  CAN3_LockSetting : Outport
  wires:
  Data Type Conversion/1 -> CAN3_LockSetting/1
  LockSetting/1 -> Data Type Conversion/1

== system halout/HAL_OUT/CAN3/FD3_BCM1_0x216/MirrorCtrl ==
  MirrorCtrl : Inport
  Data Type Conversion : DataTypeConversion  OutDataTypeStr=uint8  RndMeth=Round
  CAN3_MirrorCtrl : Outport
  wires:
  Data Type Conversion/1 -> CAN3_MirrorCtrl/1
  MirrorCtrl/1 -> Data Type Conversion/1

== system halout/HAL_OUT/CAN3/FD3_BCM1_0x216/MirrorDefog ==
  MirrorDefog : Inport
  Data Type Conversion : DataTypeConversion  OutDataTypeStr=uint8  RndMeth=Round
  CAN3_MirrorDefog : Outport
  wires:
  Data Type Conversion/1 -> CAN3_MirrorDefog/1
  MirrorDefog/1 -> Data Type Conversion/1

== system halout/HAL_OUT/CAN3/FD3_BCM1_0x216/PosLamp ==
  PosLamp : Inport
  Data Type Conversion : DataTypeConversion  OutDataTypeStr=uint8  RndMeth=Round
  CAN3_PosLamp : Outport
  wires:
  Data Type Conversion/1 -> CAN3_PosLamp/1
  PosLamp/1 -> Data Type Conversion/1

== system halout/HAL_OUT/CAN3/FD3_BCM1_0x216/PsDoorSW ==
  PsDoorSW : Inport
  Data Type Conversion : DataTypeConversion  OutDataTypeStr=uint8  RndMeth=Round
  CAN3_PsDoorSW : Outport
  wires:
  Data Type Conversion/1 -> CAN3_PsDoorSW/1
  PsDoorSW/1 -> Data Type Conversion/1

== system halout/HAL_OUT/CAN3/FD3_BCM1_0x216/RBSD ==
  RBSD : Inport
  Data Type Conversion : DataTypeConversion  OutDataTypeStr=uint8  RndMeth=Round
  CAN3_RBSD : Outport
  wires:
  Data Type Conversion/1 -> CAN3_RBSD/1
  RBSD/1 -> Data Type Conversion/1

== system halout/HAL_OUT/CAN3/FD3_BCM1_0x216/RDRL ==
  RDRL : Inport
  Data Type Conversion : DataTypeConversion  OutDataTypeStr=uint8  RndMeth=Round
  CAN3_RDRL : Outport
  wires:
  Data Type Conversion/1 -> CAN3_RDRL/1
  RDRL/1 -> Data Type Conversion/1

== system halout/HAL_OUT/CAN3/FD3_BCM1_0x216/RLDoorSW ==
  RLDoorSW : Inport
  Data Type Conversion : DataTypeConversion  OutDataTypeStr=uint8  RndMeth=Round
  CAN3_RLDoorSW : Outport
  wires:
  Data Type Conversion/1 -> CAN3_RLDoorSW/1
  RLDoorSW/1 -> Data Type Conversion/1

== system halout/HAL_OUT/CAN3/FD3_BCM1_0x216/RRDoorSW ==
  RRDoorSW : Inport
  Data Type Conversion : DataTypeConversion  OutDataTypeStr=uint8  RndMeth=Round
  CAN3_RRDoorSW : Outport
  wires:
  Data Type Conversion/1 -> CAN3_RRDoorSW/1
  RRDoorSW/1 -> Data Type Conversion/1

== system halout/HAL_OUT/CAN3/FD3_BCM1_0x216/RTurnLP ==
  RTurnLP : Inport
  Data Type Conversion : DataTypeConversion  OutDataTypeStr=uint8  RndMeth=Round
  CAN3_RTurnLP : Outport
  wires:
  Data Type Conversion/1 -> CAN3_RTurnLP/1
  RTurnLP/1 -> Data Type Conversion/1

== system halout/HAL_OUT/CAN3/FD3_BCM1_0x216/ReverseLamp ==
  ReverseLamp : Inport
  Data Type Conversion : DataTypeConversion  OutDataTypeStr=uint8  RndMeth=Round
  CAN3_ReverseLamp : Outport
  wires:
  Data Type Conversion/1 -> CAN3_ReverseLamp/1
  ReverseLamp/1 -> Data Type Conversion/1

== system halout/HAL_OUT/CAN3/FD3_BCM1_0x216/RoomLampH ==
  RoomLampH : Inport
  Data Type Conversion : DataTypeConversion  OutDataTypeStr=uint8  RndMeth=Round
  CAN3_RoomLampH : Outport
  wires:
  Data Type Conversion/1 -> CAN3_RoomLampH/1
  RoomLampH/1 -> Data Type Conversion/1

== system halout/HAL_OUT/CAN3/FD3_BCM1_0x216/RoomLampL ==
  RoomLampL : Inport
  Data Type Conversion : DataTypeConversion  OutDataTypeStr=uint8  RndMeth=Round
  CAN3_RoomLampL : Outport
  wires:
  Data Type Conversion/1 -> CAN3_RoomLampL/1
  RoomLampL/1 -> Data Type Conversion/1

== system halout/HAL_OUT/CAN3/FD3_BCM1_0x216/RrChargingDoorCtrl ==
  RrChargingDoorCtrl : Inport
  Data Type Conversion : DataTypeConversion  OutDataTypeStr=uint8  RndMeth=Round
  CAN3_Rr_ChargingDoorCtrl : Outport
  wires:
  Data Type Conversion/1 -> CAN3_Rr_ChargingDoorCtrl/1
  RrChargingDoorCtrl/1 -> Data Type Conversion/1

== system halout/HAL_OUT/CAN3/FD3_BCM1_0x216/RrDefog ==
  RrDefog : Inport
  Data Type Conversion : DataTypeConversion  OutDataTypeStr=uint8  RndMeth=Round
  CAN3_Rr_Defog : Outport
  wires:
  Data Type Conversion/1 -> CAN3_Rr_Defog/1
  RrDefog/1 -> Data Type Conversion/1

== system halout/HAL_OUT/CAN3/FD3_BCM1_0x216/RrFogLamp ==
  RrFogLamp : Inport
  Data Type Conversion : DataTypeConversion  OutDataTypeStr=uint8  RndMeth=Round
  CAN3_Rr_FogLamp : Outport
  wires:
  Data Type Conversion/1 -> CAN3_Rr_FogLamp/1
  RrFogLamp/1 -> Data Type Conversion/1

== system halout/HAL_OUT/CAN3/FD3_BCM1_0x216/RrWiper ==
  RrWiper : Inport
  Data Type Conversion : DataTypeConversion  OutDataTypeStr=uint8  RndMeth=Round
  CAN3_Rr_Wiper : Outport
  wires:
  Data Type Conversion/1 -> CAN3_Rr_Wiper/1
  RrWiper/1 -> Data Type Conversion/1

== system halout/HAL_OUT/CAN3/FD3_BCM1_0x216/TailgateHDSW ==
  TailgateHDSW : Inport
  Data Type Conversion : DataTypeConversion  OutDataTypeStr=uint8  RndMeth=Round
  CAN3_TailgateHDSW : Outport
  wires:
  Data Type Conversion/1 -> CAN3_TailgateHDSW/1
  TailgateHDSW/1 -> Data Type Conversion/1

== system halout/HAL_OUT/CAN3/FD3_BCM1_0x216/TailgateRemote ==
  TailgateRemote : Inport
  Data Type Conversion : DataTypeConversion  OutDataTypeStr=uint8  RndMeth=Round
  CAN3_TailgateRemote : Outport
  wires:
  Data Type Conversion/1 -> CAN3_TailgateRemote/1
  TailgateRemote/1 -> Data Type Conversion/1

== system halout/HAL_OUT/CAN3/FD3_BCM1_0x216/TailgateSW ==
  TailgateSW : Inport
  Data Type Conversion : DataTypeConversion  OutDataTypeStr=uint8  RndMeth=Round
  CAN3_Tailgate_SW : Outport
  wires:
  Data Type Conversion/1 -> CAN3_Tailgate_SW/1
  TailgateSW/1 -> Data Type Conversion/1

== system halout/HAL_OUT/CAN3/FD3_BCM1_0x216/TrunkRel ==
  TrunkRel : Inport
  Data Type Conversion : DataTypeConversion  OutDataTypeStr=uint8  RndMeth=Round
  CAN3_TrunkRel : Outport
  wires:
  Data Type Conversion/1 -> CAN3_TrunkRel/1
  TrunkRel/1 -> Data Type Conversion/1

== system halout/HAL_OUT/CAN3/FD3_BCM1_0x216/WasherCtrl ==
  WasherCtrl : Inport
  Data Type Conversion : DataTypeConversion  OutDataTypeStr=uint8  RndMeth=Round
  CAN3_WasherCtrl : Outport
  wires:
  Data Type Conversion/1 -> CAN3_WasherCtrl/1
  WasherCtrl/1 -> Data Type Conversion/1

== system halout/HAL_OUT/CAN3/FD3_BCM1_0x216/WiperFixMode ==
  WiperFixMode : Inport
  Data Type Conversion : DataTypeConversion  OutDataTypeStr=uint8  RndMeth=Round
  CAN3_WiperFixMode : Outport
  wires:
  Data Type Conversion/1 -> CAN3_WiperFixMode/1
  WiperFixMode/1 -> Data Type Conversion/1

== system halout/HAL_OUT/CAN3/FD3_THCM1_0x182/BatteryMode ==
  BatteryMode : Inport
  Data Type Conversion : DataTypeConversion  OutDataTypeStr=uint8  RndMeth=Round
  CAN3_BatteryMode : Outport
  wires:
  Data Type Conversion/1 -> CAN3_BatteryMode/1
  BatteryMode/1 -> Data Type Conversion/1

== system halout/HAL_OUT/CAN3/FD3_THCM1_0x182/CCUACLampSts ==
  CCUACLampSts : Inport
  Data Type Conversion : DataTypeConversion  OutDataTypeStr=uint8  RndMeth=Round
  CAN3_CCU_ACLampSts : Outport
  wires:
  Data Type Conversion/1 -> CAN3_CCU_ACLampSts/1
  CCUACLampSts/1 -> Data Type Conversion/1

== system halout/HAL_OUT/CAN3/FD3_THCM1_0x182/CCUACMaxLampSts ==
  CCUACMaxLampSts : Inport
  Data Type Conversion : DataTypeConversion  OutDataTypeStr=uint8  RndMeth=Round
  CAN3_CCU_ACMaxLampSts : Outport
  wires:
  Data Type Conversion/1 -> CAN3_CCU_ACMaxLampSts/1
  CCUACMaxLampSts/1 -> Data Type Conversion/1

== system halout/HAL_OUT/CAN3/FD3_THCM1_0x182/CCUAutoLampSts ==
  CCUAutoLampSts : Inport
  Data Type Conversion : DataTypeConversion  OutDataTypeStr=uint8  RndMeth=Round
  CAN3_CCU_AutoLampSts : Outport
  wires:
  Data Type Conversion/1 -> CAN3_CCU_AutoLampSts/1
  CCUAutoLampSts/1 -> Data Type Conversion/1

== system halout/HAL_OUT/CAN3/FD3_THCM1_0x182/CCUAutoMidLampSts ==
  CCUAutoMidLampSts : Inport
  Data Type Conversion : DataTypeConversion  OutDataTypeStr=uint8  RndMeth=Round
  CAN3_CCU_AutoMidLampSts : Outport
  wires:
  Data Type Conversion/1 -> CAN3_CCU_AutoMidLampSts/1
  CCUAutoMidLampSts/1 -> Data Type Conversion/1

== system halout/HAL_OUT/CAN3/FD3_THCM1_0x182/CCUDispalyRequest ==
  CCUDispalyRequest : Inport
  Data Type Conversion : DataTypeConversion  OutDataTypeStr=uint8  RndMeth=Round
  CAN3_CCU_Dispaly_Request : Outport
  wires:
  Data Type Conversion/1 -> CAN3_CCU_Dispaly_Request/1
  CCUDispalyRequest/1 -> Data Type Conversion/1

== system halout/HAL_OUT/CAN3/FD3_THCM1_0x182/CCUEcoSts ==
  CCUEcoSts : Inport
  Data Type Conversion : DataTypeConversion  OutDataTypeStr=uint8  RndMeth=Round
  CAN3_CCU_EcoSts : Outport
  wires:
  Data Type Conversion/1 -> CAN3_CCU_EcoSts/1
  CCUEcoSts/1 -> Data Type Conversion/1

== system halout/HAL_OUT/CAN3/FD3_THCM1_0x182/CCUFrtOnOffLampSts ==
  CCUFrtOnOffLampSts : Inport
  Data Type Conversion : DataTypeConversion  OutDataTypeStr=uint8  RndMeth=Round
  CAN3_CCU_FrtOnOffLampSts : Outport
  wires:
  Data Type Conversion/1 -> CAN3_CCU_FrtOnOffLampSts/1
  CCUFrtOnOffLampSts/1 -> Data Type Conversion/1

== system halout/HAL_OUT/CAN3/FD3_THCM1_0x182/CCUHEATMaxLampSts ==
  CCUHEATMaxLampSts : Inport
  Data Type Conversion : DataTypeConversion  OutDataTypeStr=uint8  RndMeth=Round
  CAN3_CCU_HEATMaxLampSts : Outport
  wires:
  Data Type Conversion/1 -> CAN3_CCU_HEATMaxLampSts/1
  CCUHEATMaxLampSts/1 -> Data Type Conversion/1

== system halout/HAL_OUT/CAN3/FD3_THCM1_0x182/CCURrOnOffLampSts ==
  CCURrOnOffLampSts : Inport
  Data Type Conversion : DataTypeConversion  OutDataTypeStr=uint8  RndMeth=Round
  CAN3_CCU_RrOnOffLampSts : Outport
  wires:
  Data Type Conversion/1 -> CAN3_CCU_RrOnOffLampSts/1
  CCURrOnOffLampSts/1 -> Data Type Conversion/1

== system halout/HAL_OUT/CAN3/FD3_THCM1_0x182/CCUSyncLampSts ==
  CCUSyncLampSts : Inport
  Data Type Conversion : DataTypeConversion  OutDataTypeStr=uint8  RndMeth=Round
  CAN3_CCU_SyncLampSts : Outport
  wires:
  Data Type Conversion/1 -> CAN3_CCU_SyncLampSts/1
  CCUSyncLampSts/1 -> Data Type Conversion/1

== system halout/HAL_OUT/CAN3/FD3_THCM1_0x182/CabinMode ==
  CabinMode : Inport
  Data Type Conversion : DataTypeConversion  OutDataTypeStr=uint8  RndMeth=Round
  CAN3_CabinMode : Outport
  wires:
  Data Type Conversion/1 -> CAN3_CabinMode/1
  CabinMode/1 -> Data Type Conversion/1

== system halout/HAL_OUT/CAN3/FD3_THCM1_0x182/EDriveMode ==
  EDriveMode : Inport
  Data Type Conversion : DataTypeConversion  OutDataTypeStr=uint8  RndMeth=Round
  CAN3_EDriveMode : Outport
  wires:
  Data Type Conversion/1 -> CAN3_EDriveMode/1
  EDriveMode/1 -> Data Type Conversion/1

== system halout/HAL_OUT/CAN3/FD3_THCM1_0x182/FDAGSCmd ==
  FDAGSCmd : Inport
  Data Type Conversion : DataTypeConversion  OutDataTypeStr=uint8  RndMeth=Round
  CAN3_FD_AGS_Cmd : Outport
  wires:
  Data Type Conversion/1 -> CAN3_FD_AGS_Cmd/1
  FDAGSCmd/1 -> Data Type Conversion/1

== system halout/HAL_OUT/CAN3/FD3_THCM1_0x182/FDRecyAutoCmd ==
  FDRecyAutoCmd : Inport
  Data Type Conversion : DataTypeConversion  OutDataTypeStr=uint8  RndMeth=Round
  CAN3_FD_RecyAuto_Cmd : Outport
  wires:
  Data Type Conversion/1 -> CAN3_FD_RecyAuto_Cmd/1
  FDRecyAutoCmd/1 -> Data Type Conversion/1

== system halout/HAL_OUT/CAN3/FD3_THCM1_0x182/FrCoolantflow ==
  FrCoolantflow : Inport
  Data Type Conversion : DataTypeConversion  OutDataTypeStr=uint8  RndMeth=Round
  convert_out : FVT_lib/hal/convert_out  gain=0.25  offset=0
  CAN3_Fr_Coolantflow : Outport
  wires:
  Data Type Conversion/1 -> CAN3_Fr_Coolantflow/1
  convert_out/1 -> Data Type Conversion/1
  FrCoolantflow/1 -> convert_out/1

== system halout/HAL_OUT/CAN3/FD3_THCM1_0x182/FrCoolanttemp ==
  FrCoolanttemp : Inport
  Data Type Conversion : DataTypeConversion  OutDataTypeStr=uint16  RndMeth=Round
  convert_out : FVT_lib/hal/convert_out  gain=1  offset=-40
  CAN3_Fr_Coolanttemp : Outport
  wires:
  Data Type Conversion/1 -> CAN3_Fr_Coolanttemp/1
  convert_out/1 -> Data Type Conversion/1
  FrCoolanttemp/1 -> convert_out/1

== system halout/HAL_OUT/CAN3/FD3_THCM1_0x182/HPThermalRecoveryReq ==
  HPThermalRecoveryReq : Inport
  Data Type Conversion : DataTypeConversion  OutDataTypeStr=uint8  RndMeth=Round
  CAN3_HPThermalRecoveryReq : Outport
  wires:
  Data Type Conversion/1 -> CAN3_HPThermalRecoveryReq/1
  HPThermalRecoveryReq/1 -> Data Type Conversion/1

== system halout/HAL_OUT/CAN3/FD3_THCM1_0x182/RrCoolantflow ==
  RrCoolantflow : Inport
  Data Type Conversion : DataTypeConversion  OutDataTypeStr=uint8  RndMeth=Round
  convert_out : FVT_lib/hal/convert_out  gain=0.25  offset=0
  CAN3_Rr_Coolantflow : Outport
  wires:
  Data Type Conversion/1 -> CAN3_Rr_Coolantflow/1
  convert_out/1 -> Data Type Conversion/1
  RrCoolantflow/1 -> convert_out/1

== system halout/HAL_OUT/CAN3/FD3_THCM1_0x182/RrCoolanttemp ==
  RrCoolanttemp : Inport
  Data Type Conversion : DataTypeConversion  OutDataTypeStr=uint16  RndMeth=Round
  convert_out : FVT_lib/hal/convert_out  gain=1  offset=-40
  CAN3_Rr_Coolanttemp : Outport
  wires:
  Data Type Conversion/1 -> CAN3_Rr_Coolanttemp/1
  convert_out/1 -> Data Type Conversion/1
  RrCoolanttemp/1 -> convert_out/1

== system halout/HAL_OUT/CAN3/FD3_THCM1_0x182/sigAirIntenZon1St ==
  sigAirIntenZon1St : Inport
  Data Type Conversion : DataTypeConversion  OutDataTypeStr=uint8  RndMeth=Round
  CAN3_sigAirIntenZon1St : Outport
  wires:
  Data Type Conversion/1 -> CAN3_sigAirIntenZon1St/1
  sigAirIntenZon1St/1 -> Data Type Conversion/1

== system halout/HAL_OUT/CAN3/FD3_THCM1_0x182/sigAirIntenZon3St ==
  sigAirIntenZon3St : Inport
  Data Type Conversion : DataTypeConversion  OutDataTypeStr=uint8  RndMeth=Round
  CAN3_sigAirIntenZon3St : Outport
  wires:
  Data Type Conversion/1 -> CAN3_sigAirIntenZon3St/1
  sigAirIntenZon3St/1 -> Data Type Conversion/1

== system halout/HAL_OUT/CAN3/FD3_THCM1_0x182/sigAmbAirT ==
  sigAmbAirT : Inport
  Data Type Conversion : DataTypeConversion  OutDataTypeStr=uint8  RndMeth=Round
  convert_out : FVT_lib/hal/convert_out  gain=0.5  offset=-40
  CAN3_sigAmbAirT : Outport
  wires:
  Data Type Conversion/1 -> CAN3_sigAmbAirT/1
  convert_out/1 -> Data Type Conversion/1
  sigAmbAirT/1 -> convert_out/1

== system halout/HAL_OUT/CAN3/FD3_THCM1_0x182/sigCbnAirT ==
  sigCbnAirT : Inport
  Data Type Conversion : DataTypeConversion  OutDataTypeStr=uint8  RndMeth=Round
  convert_out : FVT_lib/hal/convert_out  gain=0.5  offset=-40
  CAN3_sigCbnAirT : Outport
  wires:
  Data Type Conversion/1 -> CAN3_sigCbnAirT/1
  convert_out/1 -> Data Type Conversion/1
  sigCbnAirT/1 -> convert_out/1

== system halout/HAL_OUT/CAN3/FD3_THCM1_0x182/sigCbnPTCPwrAct ==
  sigCbnPTCPwrAct : Inport
  Data Type Conversion : DataTypeConversion  OutDataTypeStr=uint8  RndMeth=Round
  convert_out : FVT_lib/hal/convert_out  gain=50  offset=0
  CAN3_sigCbnPTCPwrAct : Outport
  wires:
  Data Type Conversion/1 -> CAN3_sigCbnPTCPwrAct/1
  convert_out/1 -> Data Type Conversion/1
  sigCbnPTCPwrAct/1 -> convert_out/1

== system halout/HAL_OUT/CAN3/FD3_THCM1_0x182/sigCbnSolarLeft ==
  sigCbnSolarLeft : Inport
  Data Type Conversion : DataTypeConversion  OutDataTypeStr=uint8  RndMeth=Round
  convert_out : FVT_lib/hal/convert_out  gain=5  offset=0
  CAN3_sigCbnSolarLeft : Outport
  wires:
  Data Type Conversion/1 -> CAN3_sigCbnSolarLeft/1
  convert_out/1 -> Data Type Conversion/1
  sigCbnSolarLeft/1 -> convert_out/1

== system halout/HAL_OUT/CAN3/FD3_THCM1_0x182/sigCbnSolarRight ==
  sigCbnSolarRight : Inport
  Data Type Conversion : DataTypeConversion  OutDataTypeStr=uint8  RndMeth=Round
  convert_out : FVT_lib/hal/convert_out  gain=5  offset=0
  CAN3_sigCbnSolarRight : Outport
  wires:
  Data Type Conversion/1 -> CAN3_sigCbnSolarRight/1
  convert_out/1 -> Data Type Conversion/1
  sigCbnSolarRight/1 -> convert_out/1

== system halout/HAL_OUT/CAN3/FD3_THCM1_0x182/sigClmtCmprPwrAct ==
  sigClmtCmprPwrAct : Inport
  Data Type Conversion : DataTypeConversion  OutDataTypeStr=uint8  RndMeth=Round
  convert_out : FVT_lib/hal/convert_out  gain=50  offset=0
  CAN3_sigClmtCmprPwrAct : Outport
  wires:
  Data Type Conversion/1 -> CAN3_sigClmtCmprPwrAct/1
  convert_out/1 -> Data Type Conversion/1
  sigClmtCmprPwrAct/1 -> convert_out/1

== system halout/HAL_OUT/CAN3/FD3_THCM1_0x182/sigClntTHvBattOut ==
  sigClntTHvBattOut : Inport
  Data Type Conversion : DataTypeConversion  OutDataTypeStr=uint8  RndMeth=Round
  convert_out : FVT_lib/hal/convert_out  gain=0.5  offset=-40
  CAN3_sigClntTHvBattOut : Outport
  wires:
  Data Type Conversion/1 -> CAN3_sigClntTHvBattOut/1
  convert_out/1 -> Data Type Conversion/1
  sigClntTHvBattOut/1 -> convert_out/1

== system halout/HAL_OUT/CAN3/FD3_THCM1_0x182/sigDfrstSt ==
  sigDfrstSt : Inport
  Data Type Conversion : DataTypeConversion  OutDataTypeStr=uint8  RndMeth=Round
  CAN3_sigDfrstSt : Outport
  wires:
  Data Type Conversion/1 -> CAN3_sigDfrstSt/1
  sigDfrstSt/1 -> Data Type Conversion/1

== system halout/HAL_OUT/CAN3/FD3_THCM1_0x182/sigHvacSt ==
  sigHvacSt : Inport
  Data Type Conversion : DataTypeConversion  OutDataTypeStr=uint8  RndMeth=Round
  CAN3_sigHvacSt : Outport
  wires:
  Data Type Conversion/1 -> CAN3_sigHvacSt/1
  sigHvacSt/1 -> Data Type Conversion/1

== system halout/HAL_OUT/CAN3/FD3_THCM1_0x182/sigRecircSt ==
  sigRecircSt : Inport
  Data Type Conversion : DataTypeConversion  OutDataTypeStr=uint8  RndMeth=Round
  CAN3_sigRecircSt : Outport
  wires:
  Data Type Conversion/1 -> CAN3_sigRecircSt/1
  sigRecircSt/1 -> Data Type Conversion/1

== system halout/HAL_OUT/CAN3/FD3_THCM1_0x182/sigSetTempZon1St ==
  sigSetTempZon1St : Inport
  Data Type Conversion : DataTypeConversion  OutDataTypeStr=uint8  RndMeth=Round
  convert_out : FVT_lib/hal/convert_out  gain=0.5  offset=17
  CAN3_sigSetTempZon1St : Outport
  wires:
  Data Type Conversion/1 -> CAN3_sigSetTempZon1St/1
  convert_out/1 -> Data Type Conversion/1
  sigSetTempZon1St/1 -> convert_out/1

== system halout/HAL_OUT/CAN3/FD3_THCM1_0x182/sigSetTempZon2St ==
  sigSetTempZon2St : Inport
  Data Type Conversion : DataTypeConversion  OutDataTypeStr=uint8  RndMeth=Round
  convert_out : FVT_lib/hal/convert_out  gain=0.5  offset=17
  CAN3_sigSetTempZon2St : Outport
  wires:
  Data Type Conversion/1 -> CAN3_sigSetTempZon2St/1
  convert_out/1 -> Data Type Conversion/1
  sigSetTempZon2St/1 -> convert_out/1

== system halout/HAL_OUT/CAN3/FD3_THCM1_0x182/sigSetTempZon3St ==
  sigSetTempZon3St : Inport
  Data Type Conversion : DataTypeConversion  OutDataTypeStr=uint8  RndMeth=Round
  convert_out : FVT_lib/hal/convert_out  gain=0.5  offset=17
  CAN3_sigSetTempZon3St : Outport
  wires:
  Data Type Conversion/1 -> CAN3_sigSetTempZon3St/1
  convert_out/1 -> Data Type Conversion/1
  sigSetTempZon3St/1 -> convert_out/1
